simulink model "dspace_2019"  (R2019b)
settings: Solver=FixedStepDiscrete  StartTime=0.0  StopTime=Inf  FixedStep=1e-3  RelTol=1e-3
PostLoadFcn:
  | , if any(exist('dsrtsu_mdlpostloadfcn', 'file') ~= 0), dsrtsu_mdlpostloadfcn('Execute', bdroot); end,
undefined symbols (not defined in the file): ami, amk1_setpoints_1, amk2_setpoints_1, amk3_setpoints_1, amk4_setpoints_1, as, digital, ebs, indicator, mcu_set_dbu_indicator_points, mcu_set_ecu_indicator_points, res_ntm_node_control
libraries: rtican x63, simulink x5, rti1401lib_dio_type3 x4, simulink_extras x1
(part 3 of 16)

== system dspace_2019/GPIO TX ==
  tx_gpio4 : Inport  PortName=tx_gpio  Element=enable_inverter4
  tx_gpio1 : Inport  PortName=tx_gpio  Element=enable_inverter1
  tx_gpio2 : Inport  PortName=tx_gpio  Element=enable_inverter2
  tx_gpio3 : Inport  PortName=tx_gpio  Element=enable_inverter3
  DIO_TYPE3_BIT_OUT_CH_BL1 : rti1401lib_dio_type3/DIO_TYPE3_BIT_OUT_CH_BL1  DSProperties=struct('RTI',struct('Version',uint32(2),'BlockType',struct('isSLSource',uint8(0),'isSLSink',uint8(1),'isHWSource',uint8(0),'isHWSink',uint8(1),'isSetup',uint8(0),'isInline',uint8(1),'isNonInline',uint8(0),'isInterrupt',uint8(0),'isChannelwise',uint8(1)),'IOBoardType',{{'DS1401','STD','DIOT3'}},'UnitType','BIT','Identifier','BITOUTCH','DialogType','ML','BlockSet','NONE','SlaveProcessor','NONE'))  RTIBlockInterface=struct('InputPortsWidth',int32(1),'InputPortsActive',1,'InputPortsDataType',{{'SS_BOOLEAN'}},'InputPortsName',{{'In'}},'BlockDisplay',{{['DIO TP3 BIT OUT\n Channelwise\nModule: 1\nPort: 1\nChannel: 2'],'center'}},'IconTransparency','on','InitLevel',3,'DialogFcn','rti1401stddiot3bitoutchgui','BlockName',struct('Token',{{'DIO_TYPE3_BIT_OUT_CH_BL1'}}))  RTIBlockParameters=struct('ModuleNo',{{1,'OFF',[1 16]}},'PortNo',{{1,'OFF',[1 3]}},'ChannelNo',{{2,'OFF',[1 16]}},'OutputStateInit',{{0,'OFF',[0 1]}},'TerminationMode',{{0,'OFF',[0 1]}},'OutputStateTermValidate',{{0,'OFF',[0 1]}},'OutputStateTerm',{{0,'OFF',[0 1]}},'SupplyRailsCh',{{[1 1],'OFF',[0 1 0 1]}},'TLCFileName',{{'rti1401dio_t3_bit_out_ch','OFF',[]}},'EnableInterrupt',{{0,'OFF',[0 1]}},'TriggerEdgeType',{{1,'OFF',[1 3]}})  RTISFcnParameters=struct('ModuleNo','int32','PortNo','int16','ChannelNo','int16','SupplyRailsCh','int16','OutputStateInit','int16','TerminationMode','int16','OutputStateTermValidate','int16','OutputStateTerm','int16','TLCFileName','char','EnableInterrupt','int16','TriggerEdgeType','int32')  RTIBlockParaDefault=struct('ModuleNo',1,'PortNo',1,'ChannelNo',1,'OutputStateInit',0,'TerminationMode',0,'OutputStateTermValidate',0,'OutputStateTerm',0,'SupplyRailsCh',[1 1],'TLCFileName','rti1401dio_t3_bit_out_ch','EnableInterrupt',0,'TriggerEdgeType',1)
  DIO_TYPE3_BIT_OUT_CH_BL2 : rti1401lib_dio_type3/DIO_TYPE3_BIT_OUT_CH_BL1  DSProperties=struct('RTI',struct('Version',uint32(2),'BlockType',struct('isSLSource',uint8(0),'isSLSink',uint8(1),'isHWSource',uint8(0),'isHWSink',uint8(1),'isSetup',uint8(0),'isInline',uint8(1),'isNonInline',uint8(0),'isInterrupt',uint8(0),'isChannelwise',uint8(1)),'IOBoardType',{{'DS1401','STD','DIOT3'}},'UnitType','BIT','Identifier','BITOUTCH','DialogType','ML','BlockSet','NONE','SlaveProcessor','NONE'))  RTIBlockInterface=struct('InputPortsWidth',int32(1),'InputPortsActive',1,'InputPortsDataType',{{'SS_BOOLEAN'}},'InputPortsName',{{'In'}},'BlockDisplay',{{['DIO TP3 BIT OUT\n Channelwise\nModule: 1\nPort: 1\nChannel: 3'],'center'}},'IconTransparency','on','InitLevel',3,'DialogFcn','rti1401stddiot3bitoutchgui','BlockName',struct('Token',{{'DIO_TYPE3_BIT_OUT_CH_BL1'}}))  RTIBlockParameters=struct('ModuleNo',{{1,'OFF',[1 16]}},'PortNo',{{1,'OFF',[1 3]}},'ChannelNo',{{3,'OFF',[1 16]}},'OutputStateInit',{{0,'OFF',[0 1]}},'TerminationMode',{{0,'OFF',[0 1]}},'OutputStateTermValidate',{{0,'OFF',[0 1]}},'OutputStateTerm',{{0,'OFF',[0 1]}},'SupplyRailsCh',{{[1 1],'OFF',[0 1 0 1]}},'TLCFileName',{{'rti1401dio_t3_bit_out_ch','OFF',[]}},'EnableInterrupt',{{0,'OFF',[0 1]}},'TriggerEdgeType',{{1,'OFF',[1 3]}})  RTISFcnParameters=struct('ModuleNo','int32','PortNo','int16','ChannelNo','int16','SupplyRailsCh','int16','OutputStateInit','int16','TerminationMode','int16','OutputStateTermValidate','int16','OutputStateTerm','int16','TLCFileName','char','EnableInterrupt','int16','TriggerEdgeType','int32')  RTIBlockParaDefault=struct('ModuleNo',1,'PortNo',1,'ChannelNo',1,'OutputStateInit',0,'TerminationMode',0,'OutputStateTermValidate',0,'OutputStateTerm',0,'SupplyRailsCh',[1 1],'TLCFileName','rti1401dio_t3_bit_out_ch','EnableInterrupt',0,'TriggerEdgeType',1)
  DIO_TYPE3_BIT_OUT_CH_BL3 : rti1401lib_dio_type3/DIO_TYPE3_BIT_OUT_CH_BL1  DSProperties=struct('RTI',struct('Version',uint32(2),'BlockType',struct('isSLSource',uint8(0),'isSLSink',uint8(1),'isHWSource',uint8(0),'isHWSink',uint8(1),'isSetup',uint8(0),'isInline',uint8(1),'isNonInline',uint8(0),'isInterrupt',uint8(0),'isChannelwise',uint8(1)),'IOBoardType',{{'DS1401','STD','DIOT3'}},'UnitType','BIT','Identifier','BITOUTCH','DialogType','ML','BlockSet','NONE','SlaveProcessor','NONE'))  RTIBlockInterface=struct('InputPortsWidth',int32(1),'InputPortsActive',1,'InputPortsDataType',{{'SS_BOOLEAN'}},'InputPortsName',{{'In'}},'BlockDisplay',{{['DIO TP3 BIT OUT\n Channelwise\nModule: 1\nPort: 1\nChannel: 4'],'center'}},'IconTransparency','on','InitLevel',3,'DialogFcn','rti1401stddiot3bitoutchgui','BlockName',struct('Token',{{'DIO_TYPE3_BIT_OUT_CH_BL1'}}))  RTIBlockParameters=struct('ModuleNo',{{1,'OFF',[1 16]}},'PortNo',{{1,'OFF',[1 3]}},'ChannelNo',{{4,'OFF',[1 16]}},'OutputStateInit',{{0,'OFF',[0 1]}},'TerminationMode',{{0,'OFF',[0 1]}},'OutputStateTermValidate',{{0,'OFF',[0 1]}},'OutputStateTerm',{{0,'OFF',[0 1]}},'SupplyRailsCh',{{[1 1],'OFF',[0 1 0 1]}},'TLCFileName',{{'rti1401dio_t3_bit_out_ch','OFF',[]}},'EnableInterrupt',{{0,'OFF',[0 1]}},'TriggerEdgeType',{{1,'OFF',[1 3]}})  RTISFcnParameters=struct('ModuleNo','int32','PortNo','int16','ChannelNo','int16','SupplyRailsCh','int16','OutputStateInit','int16','TerminationMode','int16','OutputStateTermValidate','int16','OutputStateTerm','int16','TLCFileName','char','EnableInterrupt','int16','TriggerEdgeType','int32')  RTIBlockParaDefault=struct('ModuleNo',1,'PortNo',1,'ChannelNo',1,'OutputStateInit',0,'TerminationMode',0,'OutputStateTermValidate',0,'OutputStateTerm',0,'SupplyRailsCh',[1 1],'TLCFileName','rti1401dio_t3_bit_out_ch','EnableInterrupt',0,'TriggerEdgeType',1)
  DIO_TYPE3_BIT_OUT_CH_BL4 : rti1401lib_dio_type3/DIO_TYPE3_BIT_OUT_CH_BL1  DSProperties=struct('RTI',struct('Version',uint32(2),'BlockType',struct('isSLSource',uint8(0),'isSLSink',uint8(1),'isHWSource',uint8(0),'isHWSink',uint8(1),'isSetup',uint8(0),'isInline',uint8(1),'isNonInline',uint8(0),'isInterrupt',uint8(0),'isChannelwise',uint8(1)),'IOBoardType',{{'DS1401','STD','DIOT3'}},'UnitType','BIT','Identifier','BITOUTCH','DialogType','ML','BlockSet','NONE','SlaveProcessor','NONE'))  RTIBlockInterface=struct('InputPortsWidth',int32(1),'InputPortsActive',1,'InputPortsDataType',{{'SS_BOOLEAN'}},'InputPortsName',{{'In'}},'BlockDisplay',{{['DIO TP3 BIT OUT\n Channelwise\nModule: 1\nPort: 1\nChannel: 1'],'center'}},'IconTransparency','on','InitLevel',3,'DialogFcn','rti1401stddiot3bitoutchgui','BlockName',struct('Token',{{'DIO_TYPE3_BIT_OUT_CH_BL1'}}))  RTIBlockParameters=struct('ModuleNo',{{1,'OFF',[1 16]}},'PortNo',{{1,'OFF',[1 3]}},'ChannelNo',{{1,'OFF',[1 16]}},'OutputStateInit',{{0,'OFF',[0 1]}},'TerminationMode',{{0,'OFF',[0 1]}},'OutputStateTermValidate',{{0,'OFF',[0 1]}},'OutputStateTerm',{{0,'OFF',[0 1]}},'SupplyRailsCh',{{[1 1],'OFF',[0 1 0 1]}},'TLCFileName',{{'rti1401dio_t3_bit_out_ch','OFF',[]}},'EnableInterrupt',{{0,'OFF',[0 1]}},'TriggerEdgeType',{{1,'OFF',[1 3]}})  RTISFcnParameters=struct('ModuleNo','int32','PortNo','int16','ChannelNo','int16','SupplyRailsCh','int16','OutputStateInit','int16','TerminationMode','int16','OutputStateTermValidate','int16','OutputStateTerm','int16','TLCFileName','char','EnableInterrupt','int16','TriggerEdgeType','int32')  RTIBlockParaDefault=struct('ModuleNo',1,'PortNo',1,'ChannelNo',1,'OutputStateInit',0,'TerminationMode',0,'OutputStateTermValidate',0,'OutputStateTerm',0,'SupplyRailsCh',[1 1],'TLCFileName','rti1401dio_t3_bit_out_ch','EnableInterrupt',0,'TriggerEdgeType',1)
  wires:
  tx_gpio1/1 -> DIO_TYPE3_BIT_OUT_CH_BL4/1
  tx_gpio4/1 -> DIO_TYPE3_BIT_OUT_CH_BL3/1
  tx_gpio3/1 -> DIO_TYPE3_BIT_OUT_CH_BL2/1
  tx_gpio2/1 -> DIO_TYPE3_BIT_OUT_CH_BL1/1

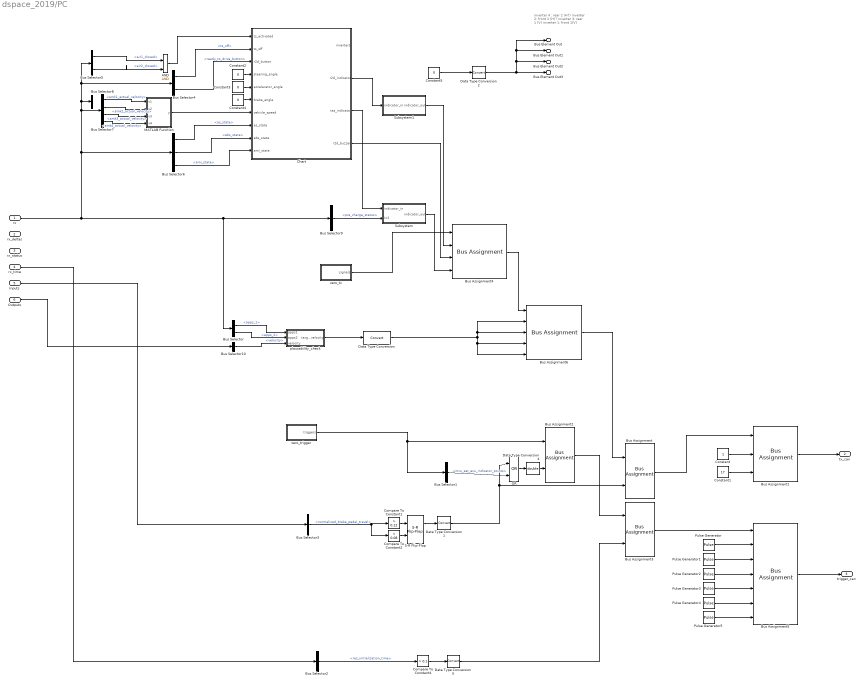
== system dspace_2019/PC ==
  note: inverter 4 : rear 2 (H?)
      | inverter 2: front 2 (H)?
      | inverter 3: rear 1 (V)
      | inverter 1: front 1(V)
  rx : Inport
  rx_deltas : Inport  Port=2
  rx_status : Inport  Port=3
  rx_time : Inport  Port=4
  Inputs : Inport  Port=5
  Outputs : Inport  Port=6
  AND : Logic  IconShape=distinctive  AllPortsSameDT=off  OutDataTypeStr=boolean
  Bus Assignment : BusAssignment  AssignedSignals=mcu_set_ecu_indicator_points.brake_light
  Bus Assignment1 : BusAssignment  AssignedSignals=res_ntm_node_control.requested_state,res_ntm_node_control.node_id
  Bus Assignment2 : BusAssignment  AssignedSignals=mcu_set_ecu_indicator_points
  Bus Assignment3 : BusAssignment  AssignedSignals=res_ntm_node_control
  Bus Assignment4 : BusAssignment  AssignedSignals=mcu_set_dbu_indicator_points.r2d_indicator_on,mcu_set_ecu_indicator_points.r2d_sound,mcu_set_dbu_indicator_points.ts_indicator_on
  Bus Assignment5 : BusAssignment  AssignedSignals=mcu_set_ecu_indicator_points,mcu_set_dbu_indicator_points,amk1_setpoints_1,amk2_setpoints_1,amk3_setpoints_1,amk4_setpoints_1
  Bus Assignment6 : BusAssignment  AssignedSignals=amk1_setpoints_1.amk1_target_velocity,amk2_setpoints_1.amk2_target_velocity,amk3_setpoints_1.amk3_target_velocity,amk4_setpoints_1.amk4_target_velocity
  Bus Selector : BusSelector  OutputSignals=dcu_pps.apps_1,dcu_pps.apps_2
  Bus Selector1 : BusSelector  OutputSignals=mcu_set_ecu_indicator_points
  Bus Selector10 : BusSelector  OutputSignals=velocity
  Bus Selector2 : BusSelector  OutputSignals=res_initialization_time
  Bus Selector3 : BusSelector  OutputSignals=normalized_brake_pedal_travel
  Bus Selector4 : BusSelector  OutputSignals=ecu_status.ts_off,dbu_status_1.ready_to_drive_button
  Bus Selector5 : BusSelector  OutputSignals=ams_status_1.air1_closed,ams_status_1.air2_closed
  Bus Selector6 : BusSelector  OutputSignals=dv_system_status.as_state,dv_system_status.ebs_state,dv_system_status.ami_state
  Bus Selector7 : BusSelector  OutputSignals=amk1_actual_values_1.amk1_actual_velocity,amk2_actual_values_1.amk2_actual_velocity,amk3_actual_values_1.amk3_actual_velocity,amk4_actual_values_1.amk4_actual_velocity
  Bus Selector8 : BusSelector  OutputSignals=dv_system_status.steering_state
  Bus Selector9 : BusSelector  OutputSignals=ams_status_1.pre_charge_status
  Chart : Stateflow chart  TreatAsAtomicUnit=on
  Compare To Constant1 : simulink/Logic and Bit Operations/Compare To Constant  relop=>  const=0.12  OutDataTypeStr=boolean
  Compare To Constant2 : simulink/Logic and Bit Operations/Compare To Constant  relop=<  const=0.08  OutDataTypeStr=boolean
  Compare To Constant4 : simulink/Logic and Bit Operations/Compare To Constant  relop=>  const=0.1  OutDataTypeStr=boolean
  Constant : Constant
  Constant1 : Constant  Value=17
  Constant{2..5} (4 alike) : Constant  Value=0
  Data Type Conversion{,1..2,5} (4 alike) : DataTypeConversion
  Data Type Conversion4 : DataTypeConversion  OutDataTypeStr=double
  MATLAB Function : MATLAB Function  TreatAsAtomicUnit=on
  OR : Logic  Operator=OR  IconShape=distinctive  AllPortsSameDT=off  OutDataTypeStr=boolean
  Pulse Generator{,1..5} (6 alike) : DiscretePulseGenerator  PulseType=Time based  Period=0.02  PulseWidth=50
  S-R Flip-Flop : simulink_extras/Flip Flops/S-R Flip-Flop  initial_condition=0
  Subsystem : Subsystem
  Subsystem1 : Subsystem
  plausability_check : Subsystem
  zero_trigger : Subsystem
  "zero_tx " : Subsystem
  Bus Element Out : Outport  PortName=tx_gpio  Element=enable_inverter1
  Bus Element Out1 : Outport  PortName=tx_gpio  Element=enable_inverter2
  Bus Element Out2 : Outport  PortName=tx_gpio  Element=enable_inverter3
  Bus Element Out3 : Outport  PortName=tx_gpio  Element=enable_inverter4
  "tx_can " : Outport  Port=2
  trigger_can : Outport  Port=3
  wires:
  Data Type Conversion1/1 -> OR/1, Bus Assignment/2
  S-R Flip-Flop/1 -> Data Type Conversion1/1
  Compare To Constant1/1 -> S-R Flip-Flop/1
  Compare To Constant2/1 -> S-R Flip-Flop/2
  rx_time/1 -> Bus Selector2/1
  Constant5/1 -> Data Type Conversion2/1
  Bus Assignment/1 -> Bus Assignment1/1
  Bus Assignment1/1 -> "tx_can "/1
  Constant/1 -> Bus Assignment1/2
  Constant1/1 -> Bus Assignment1/3
  zero_trigger/1(triggers) -> Bus Selector1/1, Bus Assignment2/1
  Bus Assignment2/1 -> Bus Assignment3/1
  Bus Selector1/1 -> OR/2  "<mcu_set_ecu_indicator_points>"
  Bus Assignment3/1 -> Bus Assignment5/1
  OR/1 -> Data Type Conversion4/1
  Data Type Conversion4/1 -> Bus Assignment2/2
  Bus Selector2/1 -> Compare To Constant4/1  "<res_initialization_time>"
  Data Type Conversion5/1 -> Bus Assignment3/2
  Compare To Constant4/1 -> Data Type Conversion5/1
  Bus Selector3/1 -> Compare To Constant1/1, Compare To Constant2/1  "<normalized_brake_pedal_travel>"
  Inputs/1 -> Bus Selector3/1
  Bus Selector7/3 -> MATLAB Function/3(v3)  "<amk3_actual_velocity>"
  Chart/3(tsa_indicator) -> Subsystem/1(indicator_in)
  Constant3/1 -> Chart/5(accelerator_angle)
  Chart/4(r2d_buzzer) -> Bus Assignment4/3
  MATLAB Function/1(y) -> Chart/7(vehicle_speed)
  Bus Selector6/2 -> Chart/9(ebs_state)  "<ebs_state>"
  Constant2/1 -> Chart/4(steering_angle)
  Bus Selector6/1 -> Chart/8(as_state)  "<as_state>"
  Chart/2(r2d_indicator) -> Subsystem1/1(indicator_in)
  Bus Selector6/3 -> Chart/10(ami_state)  "<ami_state>"
  Bus Selector5/1 -> AND/1  "<air1_closed>"
  Subsystem1/1(indicator_out) -> Bus Assignment4/2
  Bus Selector7/4 -> MATLAB Function/4(v4)  "<amk4_actual_velocity>"
  rx/1 -> Bus Selector5/1, Bus Selector4/1, Bus Selector8/1, Bus Selector7/1, Bus Selector6/1, Bus Selector9/1, Bus Selector/1
  Bus Selector5/2 -> AND/2  "<air2_closed>"
  Bus Selector4/1 -> Chart/2(ts_off)  "<ts_off>"
  Bus Selector4/2 -> Chart/3(r2d_button)  "<ready_to_drive_button>"
  Bus Selector7/2 -> MATLAB Function/2(v2)  "<amk2_actual_velocity>"
  Bus Selector9/1 -> Subsystem/2(In2)  "<pre_charge_status>"
  Bus Selector7/1 -> MATLAB Function/1(v1)  "<amk1_actual_velocity>"
  Subsystem/1(indicator_out) -> Bus Assignment4/4
  Constant4/1 -> Chart/6(brake_angle)
  AND/1 -> Chart/1(ts_activated)
  Bus Assignment5/1 -> trigger_can/1
  Pulse Generator3/1 -> Bus Assignment5/5
  Pulse Generator2/1 -> Bus Assignment5/4
  Pulse Generator/1 -> Bus Assignment5/2
  Pulse Generator4/1 -> Bus Assignment5/6
  Pulse Generator5/1 -> Bus Assignment5/7
  Pulse Generator1/1 -> Bus Assignment5/3
  "zero_tx "/1(signals) -> Bus Assignment4/1
  Data Type Conversion2/1 -> Bus Element Out/1, Bus Element Out1/1, Bus Element Out2/1, Bus Element Out3/1
  Bus Selector/1 -> plausability_check/1(apps1)  "<apps_1>"
  Bus Selector/2 -> plausability_check/2(apps2)  "<apps_2>"
  Bus Assignment4/1 -> Bus Assignment6/1
  Data Type Conversion/1 -> Bus Assignment6/5, Bus Assignment6/4, Bus Assignment6/3, Bus Assignment6/2
  Bus Assignment6/1 -> Bus Assignment/1
  Outputs/1 -> Bus Selector10/1
  Bus Selector10/1 -> plausability_check/3(velocity)  "<velocity>"
  plausability_check/1(target_velocity) -> Data Type Conversion/1

== system dspace_2019/RTI Data ==
  RTI Data Store : Subsystem  Tag="struct('private',struct('version',struct('dsVer',uint32(2),'dsVerCreation',uint32(2),'RTI',struct('ver','7.13','type','RTI1401')),'access',struct('type','Model','isPerm',1,'created',['29-Jun-2022 11:04:06'],'modified',['25-Jul-2022 13:04:18'],'location','')),'public',struct('main',struct('data',[]),'sub',struct('name',{{'dspace'}},'data',{{struct('TH',struct('thTaskInfo',struct('taskType',{'TIMER','HWINT','TMRINT','SWINT','GLINT'},'tasksNumOf',{1,0,0,0,0},'srcIds',{{'TIMERA'},{},{},{},{}},'taskNames',{{['Timer Task 1']},{},{},{},{}})),'th_tc',struct('dataType','TASK','taskGroupId','','taskGroupList',{{}},'taskSchedulingPolicy','FCFS','taskType','TIMER','blkh',-1,'srcId','TIMERA','srcSgnName',['Timer A interrupt'],'srcCpuName','','taskName',['Timer Task 1  [0.001] s'],'taskNameDisplayExt','','smplTime',0.001,'smplTimeOffs',0,'hasFixedPriority',0,'priority',1,'hasFixedOvc',0,'ovcType',1,'ovcMax',1),'tc_th',struct('dataType','TASK','taskGroupId','','taskGroupList',{{}},'taskSchedulingPolicy','FCFS','taskType','TIMER','blkh',-1,'srcId','TIMERA','srcSgnName',['Timer A interrupt'],'srcCpuName','','taskName',['Timer Task 1  [0.001] s'],'taskNameDisplayExt','','smplTime',0.001,'smplTimeOffs',0,'hasFixedPriority',0,'priority',1,'hasFixedOvc',0,'ovcType',1,'ovcMax',1))}})))"  mask(RTI_DATA_STORE){}
      mask help:
      | RTI Data Store Block. This block is used by RTI to store internal model dependent data. Deleting this block will result in data loss.
      |
      | NEVER DELETE, COPY, OR MODIFY THIS BLOCK!
      mask Help:
      | RTI Data Store Block. This block is used by RTI to store internal model dependent data. Deleting this block will result in data loss.
      | 
      | NEVER DELETE, COPY, OR MODIFY THIS BLOCK!
      mask Display: text(0.5, 0.5, ' ', 'HorizontalAlignment', 'center');

== system dspace_2019/Signal Preconditioning ==
  rx : Inport
  rx_deltas : Inport  Port=2
  rx_status : Inport  Port=3
  rx_time : Inport  Port=4
  Bus Selector8 : BusSelector  OutputSignals=dcu_pps.bpps_1,dcu_pps.bpps_2,dcu_pps.apps_1,dcu_pps.apps_2
  Compare To Constant : simulink/Logic and Bit Operations/Compare To Constant  relop=>  const=0.1  OutDataTypeStr=boolean
  Integrator : Integrator  ExternalReset=falling
  MATLAB Function1 : MATLAB Function  TreatAsAtomicUnit=on
  MATLAB Function2 : MATLAB Function  TreatAsAtomicUnit=on
  Bus Element Out : Outport  PortName=Inputs  Element=normalized_brake_pedal_travel
  Out Bus Element : Outport  PortName=Inputs  Element=apps_implausability
  Out Bus Element1 : Outport  PortName=Inputs  Element=normalized_accelerator_pedal_travel
  wires:
  Bus Selector8/2 -> MATLAB Function1/2(bpps2)  "<bpps_2>"
  Bus Selector8/1 -> MATLAB Function1/1(bpps1)  "<bpps_1>"
  rx/1 -> Bus Selector8/1
  MATLAB Function1/1(normalized_brake_pedal_travel) -> Bus Element Out/1
  Bus Selector8/3 -> MATLAB Function2/1(apps1)  "<apps_1>"
  Bus Selector8/4 -> MATLAB Function2/2(apps2)  "<apps_2>"
  MATLAB Function2/2(implausability) -> Integrator/2, Integrator/1
  Integrator/1 -> Compare To Constant/1
  Compare To Constant/1 -> Out Bus Element/1
  MATLAB Function2/1(normalized_accelerator_pedal_travel) -> Out Bus Element1/1

== system dspace_2019/Vehicular Control ==
  rx : Inport
  Bus Element In : Inport  Port=2  PortName=Inputs  Element=normalized_brake_pedal_travel
  In Bus Element : Inport  Port=2  PortName=Inputs  Element=normalized_accelerator_pedal_travel
  Bus Selector : BusSelector  OutputSignals=dv_system_status.as_state,dv_control_target.dv_speed_target
  MATLAB Function : MATLAB Function  TreatAsAtomicUnit=on
  Out Bus Element : Outport  PortName=Outputs  Element=velocity
  wires:
  rx/1 -> Bus Selector/1
  Bus Selector/1 -> MATLAB Function/1(car_state)  "<as_state>"
  In Bus Element/1 -> MATLAB Function/3(accelerator_pedal)
  Bus Selector/2 -> MATLAB Function/2(as_speed)  "<dv_speed_target>"
  MATLAB Function/1(velocity) -> Out Bus Element/1

== system dspace_2019/CAN RX/FSE_EnergyMeter_Data ==
  FSE_EnergyMeter_Data1 : rtican/RTICAN Receive (RX)   Reserved1=[]  Reserved2=[]  Reserved3=[]  Reserved4=[]  SfcnMessage=[]  Msg_Struct=[]  BoardTypeNo=[]  BoardNo=[]  ChannelNo=[]  Parameters=[]  DialogFcn=[]  UnitName=[]  Revision=[]  UnitValues=[]  DSProperties=struct('RTI',struct('Version',uint32(5),'BlockType',struct('isSLSource',uint8(1),'isSLSink',uint8(1),'isHWSource',uint8(0),'isHWSink',uint8(0),'isSetup',uint8(0),'isInline',uint8(1),'isNonInline',uint8(0),'isInterrupt',uint8(0),'isChannelwise',uint8(0)),'IOBoardType','RTICAN','UnitType','MESSAGE','Identifier','RX','DialogType','MSVC','BlockSet','RTICAN','SlaveProcessor','CAN'))  RTIBlockInterface=struct('OutputPortsWidth',int32([1 1 1 1 1 1 1 1]),'OutputPortsActive',[1 1 1 1 1 1 1 1],'OutputPortsName',{{'MsgCntr','Status','Power','Voltage','Current',['RX status'],['RX time'],['RX delta time']}},'OutputPortsDataType',{{'SS_DOUBLE','SS_DOUBLE','SS_DOUBLE','SS_DOUBLE','SS_DOUBLE','SS_DOUBLE','SS_DOUBLE','SS_DOUBLE'}},'OutputPortsLabel',{{'MsgCntr','Status','Power','Voltage','Current','','',''}},'OutputPortsLabelMode','ON','InputPortsWidth',int32(0),'InputPortsActive',0,'DialogFcn','rtican_message_interface_gui','BlockDisplay',{{'','center'}},'IconTransparency','on','ParameterTunableNames',{{}},'InitLevel',3,'BlockName',struct('Token',{{'FSE_EnergyMeter_Data'}}),'SampleTime',{{-1}},'TriggerPort',{{'none'}},'EnablePort',{{'none'}})  RTIBlockParameters=struct('BoardTypeNo',{{1,'OFF',[]}},'BoardNo',{{1,'ON',[1 16]}},'ChannelNo',{{2,'ON',[1 2]}},'Parameters',{{struct('DataFileSupport',struct('DataFileSelectedMaster',1,'DataFileSelectedLocal',1,'DataFileName','c:\users\oscar\documents\github\sw_infrastructure\kthfspe_python\databases\can1.dbc|','DataFileDate',{{{['10-Jul-2022 16:14:04']}}},'SelectedFile','c:\users\oscar\documents\github\sw_infrastructure\kthfspe_python\databases\can1.dbc'),'Options',struct('StatusSelected',1,'TimeSelected',1,'DeltaTimeSelected',1,'BytePortSelected',0,'MessageLengthSelected',0,'TriggerPort',struct('Selected',0,'TriggerType',0),'UserCoding',struct('Selected',0,'InterfaceFile','UserDecodingFile','FcnName','UserDecodeFcn','InportSelected',0,'InportWidth',1,'OutportSelected',0,'OutportWidth',1),'EnablePortSelected',0,'SignalOnPortnameSelected',1,'UseRXService',0),'Message',struct('MsgOnBlocknameSelected',1,'MsgName','FSE_EnergyMeter_Data','MsgIdFormat',0,'MsgId',1072,'MsgLength',8,'NumSignals',5,'SampleTime',-1,'Signal',struct('SgnName',{'MsgCntr','Status','Power','Voltage','Current'},'SgnStartBit',{0,8,16,32,48},'SgnLength',{8,8,16,16,16},'SgnType',{0,0,0,0,0},'ModeValue',{-1,-1,-1,-1,-1},'DataType',{0,0,1,1,1},'ByteLayout',{0,0,0,0,0},'Factor',{1,1,3,0.04,0.05},'Offset',{0,0,0,0,0},'SgnComment',{{''},{''},{''},{''},{''}},'SgnUnit',{'','','W','V','A'},'Min',{0,0,-98304,-1310.72,-1638.4},'Max',{255,255,98301,1310.68,1638.35},'SLDataType',{'SS_DOUBLE','SS_DOUBLE','SS_DOUBLE','SS_DOUBLE','SS_DOUBLE'}),'MsgIdNumFormat',0,'MsgComment',{{''}}),'Version',1.2,'general',struct('isFromLib',0)),'OFF',[]}},'GroupId',{{struct('Group',{{'RTICAN'}},'No',1,'Behavior',{{'NAMECHANGE'}},'BlockType',{{'SINK'}},'NameChangeFlag',0),'OFF',[]}},'SFcnRTICANMessage',{{struct('MsgType','RX','SFcnPortType','Scalar','MsgName','FSE_EnergyMeter_Data','MsgIdFormat','STD','MsgId',1072,'MsgLength',8,'NumSignals',5,'SampleTime',-1,'Signal',struct('SgnName',{'MsgCntr','Status','Power','Voltage','Current'},'SgnStartBit',{0,8,16,32,48},'SgnLength',{8,8,16,16,16},'SgnType',{'standard','standard','standard','standard','standard'},'ModeValue',{-1,-1,-1,-1,-1},'DataType',{['unsigned int'],['unsigned int'],['signed int'],['signed int'],['signed int']},'ByteLayout',{['little endian'],['little endian'],['little endian'],['little endian'],['little endian']},'Factor',{1,1,3,0.04,0.05},'Offset',{0,0,0,0,0},'SLDataType',{'SS_DOUBLE','SS_DOUBLE','SS_DOUBLE','SS_DOUBLE','SS_DOUBLE'}),'StatusSelected','yes','TimeSelected','yes','DeltaTimeSelected','yes','BytePortSelected','no','MessageLengthSelected','no','TriggerPort',struct('Selected','no','TriggerType',0),'UserCoding',struct('Selected','no','InterfaceFile','UserDecodingFile','FcnName','UserDecodeFcn','InportSelected','no','InportWidth',1,'OutportSelected','no','OutportWidth',1),'EnablePortSelected','no','UseRXService','no','BoardType','DS1','BoardNo',1,'ControllerNo',1),'OFF',[]}},'TLCFileName',{{'rtican_rx_message','OFF',[]}})  RTISFcnParameters=struct('SFcnRTICANMessage','struct','TLCFileName','char')  RTIBlockParaDefault=struct('BoardTypeNo',4302,'BoardNo',1,'ChannelNo',1,'Parameters',struct('DataFileSupport',struct('DataFileSelectedMaster',0,'DataFileSelectedLocal',0,'DataFileName','','DataFileDate','','SelectedFile',['<no file selected>']),'Options',struct('StatusSelected',1,'TimeSelected',1,'DeltaTimeSelected',1,'BytePortSelected',0,'MessageLengthSelected',0,'TriggerPort',struct('Selected',0,'TriggerType','rising'),'UserCoding',struct('Selected',0,'InterfaceFile','UserDecodingFile','FcnName','UserDecodeFcn','InportSelected',0,'InportWidth',1,'OutportSelected',0,'OutportWidth',1),'EnablePortSelected',0,'SignalOnPortnameSelected',1,'UseRXService',0),'Message',struct('MsgOnBlocknameSelected',0,'MsgName',['RX Message'],'MsgIdFormat',0,'MsgId',100,'MsgLength',8,'NumSignals',1,'SampleTime',-1,'Signal',struct('SgnName',['RX signal'],'SgnStartBit',0,'SgnLength',8,'SgnType',0,'ModeValue',-1,'DataType',0,'SLDataType','SS_DOUBLE','ByteLayout',0,'Factor',1,'Offset',0,'Min',0,'Max',255,'SgnComment',{{}},'SgnUnit',''),'MsgIdNumFormat',0,'MsgComment',{{''}}),'Version',1.2,'general',struct('isFromLib',1)),'GroupId',struct('Group',{{'RTICAN'}},'No',1,'Behavior',{{'NAMECHANGE'}},'BlockType',{{'SINK'}},'NameChangeFlag',0),'SFcnRTICANMessage',struct('MsgType','RX','MsgName',['RX Message'],'MsgIdFormat','STD','MsgId',100,'MsgLength',8,'NumSignals',1,'SampleTime',-1,'Signal',struct('SgnName',['RX signal'],'SgnStartBit',0,'SgnLength',8,'SgnType','standard','ModeValue',-1,'DataType',['unsigned int'],'ByteLayout',['little endian'],'SLDataType','SS_DOUBLE','Factor',1,'Offset',0),'StatusSelected','yes','TimeSelected','yes','DeltaTimeSelected','yes','BytePortSelected','no','MessageLengthSelected','no','EnablePortSelected','no','UserCoding',struct('Selected','no','InterfaceFile','UserDecodingFile','FcnName','UserDecodeFcn','InportSelected','no','InportWidth',1,'OutportSelected','no','OutportWidth',1),'TriggerPort',struct('Selected','no','TriggerType','rising'),'UseRXService','no','BoardType','DS4302','BoardNo',1,'ControllerNo',1,'SFcnPortType','Scalar'),'TLCFileName','rtican_rx_message')
      settings: AttributesFormatString=Group Id: RTICAN1\n  SourceProductName=dSPACE RTI CAN Blockset
  clock_time : Clock
  sub_time : Sum  Inputs=+-
  MsgCntr_bus : Outport  PortName=signals  Element=MsgCntr
  Status_bus : Outport  PortName=signals  Element=Status
  Power_bus : Outport  PortName=signals  Element=Power
  Voltage_bus : Outport  PortName=signals  Element=Voltage
  Current_bus : Outport  PortName=signals  Element=Current
  status : Outport  Port=2
  time : Outport  Port=3
  delta : Outport  Port=4
  wires:
  clock_time/1 -> sub_time/1
  sub_time/1 -> time/1
  FSE_EnergyMeter_Data1/6 -> status/1
  FSE_EnergyMeter_Data1/7 -> sub_time/2
  FSE_EnergyMeter_Data1/8 -> delta/1
  FSE_EnergyMeter_Data1/1 -> MsgCntr_bus/1  "MsgCntr"
  FSE_EnergyMeter_Data1/2 -> Status_bus/1  "Status"
  FSE_EnergyMeter_Data1/3 -> Power_bus/1  "Power"
  FSE_EnergyMeter_Data1/4 -> Voltage_bus/1  "Voltage"
  FSE_EnergyMeter_Data1/5 -> Current_bus/1  "Current"

== system dspace_2019/CAN RX/SBG_ECAN_MSG_AUTO_SLIP_CURV ==
  SBG_ECAN_MSG_AUTO_SLIP_CURV1 : rtican/RTICAN Receive (RX)   Reserved1=[]  Reserved2=[]  Reserved3=[]  Reserved4=[]  SfcnMessage=[]  Msg_Struct=[]  BoardTypeNo=[]  BoardNo=[]  ChannelNo=[]  Parameters=[]  DialogFcn=[]  UnitName=[]  Revision=[]  UnitValues=[]  DSProperties=struct('RTI',struct('Version',uint32(5),'BlockType',struct('isSLSource',uint8(1),'isSLSink',uint8(1),'isHWSource',uint8(0),'isHWSink',uint8(0),'isSetup',uint8(0),'isInline',uint8(1),'isNonInline',uint8(0),'isInterrupt',uint8(0),'isChannelwise',uint8(0)),'IOBoardType','RTICAN','UnitType','MESSAGE','Identifier','RX','DialogType','MSVC','BlockSet','RTICAN','SlaveProcessor','CAN'))  RTIBlockInterface=struct('OutputPortsWidth',int32([1 1 1 1 1 1 1]),'OutputPortsActive',[1 1 1 1 1 1 1],'OutputPortsName',{{'ANGLE_TRACK','ANGLE_SLIP','CURVATURE_RADIUS','AUTO_STATUS',['RX status'],['RX time'],['RX delta time']}},'OutputPortsDataType',{{'SS_DOUBLE','SS_DOUBLE','SS_DOUBLE','SS_DOUBLE','SS_DOUBLE','SS_DOUBLE','SS_DOUBLE'}},'OutputPortsLabel',{{'ANGLE_TRACK','ANGLE_SLIP','CURVATURE_RADIUS','AUTO_STATUS','','',''}},'OutputPortsLabelMode','ON','InputPortsWidth',int32(0),'InputPortsActive',0,'DialogFcn','rtican_message_interface_gui','BlockDisplay',{{'','center'}},'IconTransparency','on','ParameterTunableNames',{{}},'InitLevel',3,'BlockName',struct('Token',{{'SBG_ECAN_MSG_AUTO_SLIP_CURV'}}),'SampleTime',{{-1}},'TriggerPort',{{'none'}},'EnablePort',{{'none'}})  RTIBlockParameters=struct('BoardTypeNo',{{1,'OFF',[]}},'BoardNo',{{1,'ON',[1 16]}},'ChannelNo',{{2,'ON',[1 2]}},'Parameters',{{struct('DataFileSupport',struct('DataFileSelectedMaster',1,'DataFileSelectedLocal',1,'DataFileName','c:\users\oscar\documents\github\sw_infrastructure\kthfspe_python\databases\can1.dbc|','DataFileDate',{{{['10-Jul-2022 16:14:04']}}},'SelectedFile','c:\users\oscar\documents\github\sw_infrastructure\kthfspe_python\databases\can1.dbc'),'Options',struct('StatusSelected',1,'TimeSelected',1,'DeltaTimeSelected',1,'BytePortSelected',0,'MessageLengthSelected',0,'TriggerPort',struct('Selected',0,'TriggerType',0),'UserCoding',struct('Selected',0,'InterfaceFile','UserDecodingFile','FcnName','UserDecodeFcn','InportSelected',0,'InportWidth',1,'OutportSelected',0,'OutportWidth',1),'EnablePortSelected',0,'SignalOnPortnameSelected',1,'UseRXService',0),'Message',struct('MsgOnBlocknameSelected',1,'MsgName','SBG_ECAN_MSG_AUTO_SLIP_CURV','MsgIdFormat',0,'MsgId',544,'MsgLength',7,'NumSignals',4,'SampleTime',-1,'Signal',struct('SgnName',{'ANGLE_TRACK','ANGLE_SLIP','CURVATURE_RADIUS','AUTO_STATUS'},'SgnStartBit',{0,16,32,48},'SgnLength',{16,16,16,8},'SgnType',{0,0,0,0},'ModeValue',{-1,-1,-1,-1},'DataType',{1,1,0,0},'ByteLayout',{0,0,0,0},'Factor',{0.0001,0.0001,0.01,1},'Offset',{0,0,0,0},'SgnComment',{{''},{''},{''},{''}},'SgnUnit',{'rad','rad','m',''},'Min',{-3.2768,-3.2768,0,0},'Max',{3.2767,3.2767,655.35,255},'SLDataType',{'SS_DOUBLE','SS_DOUBLE','SS_DOUBLE','SS_DOUBLE'}),'MsgIdNumFormat',0,'MsgComment',{{''}}),'Version',1.2,'general',struct('isFromLib',0)),'OFF',[]}},'GroupId',{{struct('Group',{{'RTICAN'}},'No',1,'Behavior',{{'NAMECHANGE'}},'BlockType',{{'SINK'}},'NameChangeFlag',0),'OFF',[]}},'SFcnRTICANMessage',{{struct('MsgType','RX','SFcnPortType','Scalar','MsgName','SBG_ECAN_MSG_AUTO_SLIP_CURV','MsgIdFormat','STD','MsgId',544,'MsgLength',7,'NumSignals',4,'SampleTime',-1,'Signal',struct('SgnName',{'ANGLE_TRACK','ANGLE_SLIP','CURVATURE_RADIUS','AUTO_STATUS'},'SgnStartBit',{0,16,32,48},'SgnLength',{16,16,16,8},'SgnType',{'standard','standard','standard','standard'},'ModeValue',{-1,-1,-1,-1},'DataType',{['signed int'],['signed int'],['unsigned int'],['unsigned int']},'ByteLayout',{['little endian'],['little endian'],['little endian'],['little endian']},'Factor',{0.0001,0.0001,0.01,1},'Offset',{0,0,0,0},'SLDataType',{'SS_DOUBLE','SS_DOUBLE','SS_DOUBLE','SS_DOUBLE'}),'StatusSelected','yes','TimeSelected','yes','DeltaTimeSelected','yes','BytePortSelected','no','MessageLengthSelected','no','TriggerPort',struct('Selected','no','TriggerType',0),'UserCoding',struct('Selected','no','InterfaceFile','UserDecodingFile','FcnName','UserDecodeFcn','InportSelected','no','InportWidth',1,'OutportSelected','no','OutportWidth',1),'EnablePortSelected','no','UseRXService','no','BoardType','DS1','BoardNo',1,'ControllerNo',1),'OFF',[]}},'TLCFileName',{{'rtican_rx_message','OFF',[]}})  RTISFcnParameters=struct('SFcnRTICANMessage','struct','TLCFileName','char')  RTIBlockParaDefault=struct('BoardTypeNo',4302,'BoardNo',1,'ChannelNo',1,'Parameters',struct('DataFileSupport',struct('DataFileSelectedMaster',0,'DataFileSelectedLocal',0,'DataFileName','','DataFileDate','','SelectedFile',['<no file selected>']),'Options',struct('StatusSelected',1,'TimeSelected',1,'DeltaTimeSelected',1,'BytePortSelected',0,'MessageLengthSelected',0,'TriggerPort',struct('Selected',0,'TriggerType','rising'),'UserCoding',struct('Selected',0,'InterfaceFile','UserDecodingFile','FcnName','UserDecodeFcn','InportSelected',0,'InportWidth',1,'OutportSelected',0,'OutportWidth',1),'EnablePortSelected',0,'SignalOnPortnameSelected',1,'UseRXService',0),'Message',struct('MsgOnBlocknameSelected',0,'MsgName',['RX Message'],'MsgIdFormat',0,'MsgId',100,'MsgLength',8,'NumSignals',1,'SampleTime',-1,'Signal',struct('SgnName',['RX signal'],'SgnStartBit',0,'SgnLength',8,'SgnType',0,'ModeValue',-1,'DataType',0,'SLDataType','SS_DOUBLE','ByteLayout',0,'Factor',1,'Offset',0,'Min',0,'Max',255,'SgnComment',{{}},'SgnUnit',''),'MsgIdNumFormat',0,'MsgComment',{{''}}),'Version',1.2,'general',struct('isFromLib',1)),'GroupId',struct('Group',{{'RTICAN'}},'No',1,'Behavior',{{'NAMECHANGE'}},'BlockType',{{'SINK'}},'NameChangeFlag',0),'SFcnRTICANMessage',struct('MsgType','RX','MsgName',['RX Message'],'MsgIdFormat','STD','MsgId',100,'MsgLength',8,'NumSignals',1,'SampleTime',-1,'Signal',struct('SgnName',['RX signal'],'SgnStartBit',0,'SgnLength',8,'SgnType','standard','ModeValue',-1,'DataType',['unsigned int'],'ByteLayout',['little endian'],'SLDataType','SS_DOUBLE','Factor',1,'Offset',0),'StatusSelected','yes','TimeSelected','yes','DeltaTimeSelected','yes','BytePortSelected','no','MessageLengthSelected','no','EnablePortSelected','no','UserCoding',struct('Selected','no','InterfaceFile','UserDecodingFile','FcnName','UserDecodeFcn','InportSelected','no','InportWidth',1,'OutportSelected','no','OutportWidth',1),'TriggerPort',struct('Selected','no','TriggerType','rising'),'UseRXService','no','BoardType','DS4302','BoardNo',1,'ControllerNo',1,'SFcnPortType','Scalar'),'TLCFileName','rtican_rx_message')
      settings: AttributesFormatString=Group Id: RTICAN1\n  SourceProductName=dSPACE RTI CAN Blockset
  clock_time : Clock
  sub_time : Sum  Inputs=+-
  ANGLE_TRACK_bus : Outport  PortName=signals  Element=ANGLE_TRACK
  ANGLE_SLIP_bus : Outport  PortName=signals  Element=ANGLE_SLIP
  CURVATURE_RADIUS_bus : Outport  PortName=signals  Element=CURVATURE_RADIUS
  AUTO_STATUS_bus : Outport  PortName=signals  Element=AUTO_STATUS
  status : Outport  Port=2
  time : Outport  Port=3
  delta : Outport  Port=4
  wires:
  clock_time/1 -> sub_time/1
  sub_time/1 -> time/1
  SBG_ECAN_MSG_AUTO_SLIP_CURV1/5 -> status/1
  SBG_ECAN_MSG_AUTO_SLIP_CURV1/6 -> sub_time/2
  SBG_ECAN_MSG_AUTO_SLIP_CURV1/7 -> delta/1
  SBG_ECAN_MSG_AUTO_SLIP_CURV1/1 -> ANGLE_TRACK_bus/1  "ANGLE_TRACK"
  SBG_ECAN_MSG_AUTO_SLIP_CURV1/2 -> ANGLE_SLIP_bus/1  "ANGLE_SLIP"
  SBG_ECAN_MSG_AUTO_SLIP_CURV1/3 -> CURVATURE_RADIUS_bus/1  "CURVATURE_RADIUS"
  SBG_ECAN_MSG_AUTO_SLIP_CURV1/4 -> AUTO_STATUS_bus/1  "AUTO_STATUS"

== system dspace_2019/CAN RX/SBG_ECAN_MSG_EKF_EULER ==
  SBG_ECAN_MSG_EKF_EULER1 : rtican/RTICAN Receive (RX)   Reserved1=[]  Reserved2=[]  Reserved3=[]  Reserved4=[]  SfcnMessage=[]  Msg_Struct=[]  BoardTypeNo=[]  BoardNo=[]  ChannelNo=[]  Parameters=[]  DialogFcn=[]  UnitName=[]  Revision=[]  UnitValues=[]  DSProperties=struct('RTI',struct('Version',uint32(5),'BlockType',struct('isSLSource',uint8(1),'isSLSink',uint8(1),'isHWSource',uint8(0),'isHWSink',uint8(0),'isSetup',uint8(0),'isInline',uint8(1),'isNonInline',uint8(0),'isInterrupt',uint8(0),'isChannelwise',uint8(0)),'IOBoardType','RTICAN','UnitType','MESSAGE','Identifier','RX','DialogType','MSVC','BlockSet','RTICAN','SlaveProcessor','CAN'))  RTIBlockInterface=struct('OutputPortsWidth',int32([1 1 1 1 1 1]),'OutputPortsActive',[1 1 1 1 1 1],'OutputPortsName',{{'ROLL','PITCH','YAW',['RX status'],['RX time'],['RX delta time']}},'OutputPortsDataType',{{'SS_DOUBLE','SS_DOUBLE','SS_DOUBLE','SS_DOUBLE','SS_DOUBLE','SS_DOUBLE'}},'OutputPortsLabel',{{'ROLL','PITCH','YAW','','',''}},'OutputPortsLabelMode','ON','InputPortsWidth',int32(0),'InputPortsActive',0,'DialogFcn','rtican_message_interface_gui','BlockDisplay',{{'','center'}},'IconTransparency','on','ParameterTunableNames',{{}},'InitLevel',3,'BlockName',struct('Token',{{'SBG_ECAN_MSG_EKF_EULER'}}),'SampleTime',{{-1}},'TriggerPort',{{'none'}},'EnablePort',{{'none'}})  RTIBlockParameters=struct('BoardTypeNo',{{1,'OFF',[]}},'BoardNo',{{1,'ON',[1 16]}},'ChannelNo',{{2,'ON',[1 2]}},'Parameters',{{struct('DataFileSupport',struct('DataFileSelectedMaster',1,'DataFileSelectedLocal',1,'DataFileName','c:\users\oscar\documents\github\sw_infrastructure\kthfspe_python\databases\can1.dbc|','DataFileDate',{{{['10-Jul-2022 16:14:04']}}},'SelectedFile','c:\users\oscar\documents\github\sw_infrastructure\kthfspe_python\databases\can1.dbc'),'Options',struct('StatusSelected',1,'TimeSelected',1,'DeltaTimeSelected',1,'BytePortSelected',0,'MessageLengthSelected',0,'TriggerPort',struct('Selected',0,'TriggerType',0),'UserCoding',struct('Selected',0,'InterfaceFile','UserDecodingFile','FcnName','UserDecodeFcn','InportSelected',0,'InportWidth',1,'OutportSelected',0,'OutportWidth',1),'EnablePortSelected',0,'SignalOnPortnameSelected',1,'UseRXService',0),'Message',struct('MsgOnBlocknameSelected',1,'MsgName','SBG_ECAN_MSG_EKF_EULER','MsgIdFormat',0,'MsgId',306,'MsgLength',6,'NumSignals',3,'SampleTime',-1,'Signal',struct('SgnName',{'ROLL','PITCH','YAW'},'SgnStartBit',{0,16,32},'SgnLength',{16,16,16},'SgnType',{0,0,0},'ModeValue',{-1,-1,-1},'DataType',{1,1,1},'ByteLayout',{0,0,0},'Factor',{0.0001,0.0001,0.0001},'Offset',{0,0,0},'SgnComment',{{''},{''},{''}},'SgnUnit',{'rad','rad','rad'},'Min',{-3.2768,-3.2768,-3.2768},'Max',{3.2767,3.2767,3.2767},'SLDataType',{'SS_DOUBLE','SS_DOUBLE','SS_DOUBLE'}),'MsgIdNumFormat',0,'MsgComment',{{''}}),'Version',1.2,'general',struct('isFromLib',0)),'OFF',[]}},'GroupId',{{struct('Group',{{'RTICAN'}},'No',1,'Behavior',{{'NAMECHANGE'}},'BlockType',{{'SINK'}},'NameChangeFlag',0),'OFF',[]}},'SFcnRTICANMessage',{{struct('MsgType','RX','SFcnPortType','Scalar','MsgName','SBG_ECAN_MSG_EKF_EULER','MsgIdFormat','STD','MsgId',306,'MsgLength',6,'NumSignals',3,'SampleTime',-1,'Signal',struct('SgnName',{'ROLL','PITCH','YAW'},'SgnStartBit',{0,16,32},'SgnLength',{16,16,16},'SgnType',{'standard','standard','standard'},'ModeValue',{-1,-1,-1},'DataType',{['signed int'],['signed int'],['signed int']},'ByteLayout',{['little endian'],['little endian'],['little endian']},'Factor',{0.0001,0.0001,0.0001},'Offset',{0,0,0},'SLDataType',{'SS_DOUBLE','SS_DOUBLE','SS_DOUBLE'}),'StatusSelected','yes','TimeSelected','yes','DeltaTimeSelected','yes','BytePortSelected','no','MessageLengthSelected','no','TriggerPort',struct('Selected','no','TriggerType',0),'UserCoding',struct('Selected','no','InterfaceFile','UserDecodingFile','FcnName','UserDecodeFcn','InportSelected','no','InportWidth',1,'OutportSelected','no','OutportWidth',1),'EnablePortSelected','no','UseRXService','no','BoardType','DS1','BoardNo',1,'ControllerNo',1),'OFF',[]}},'TLCFileName',{{'rtican_rx_message','OFF',[]}})  RTISFcnParameters=struct('SFcnRTICANMessage','struct','TLCFileName','char')  RTIBlockParaDefault=struct('BoardTypeNo',4302,'BoardNo',1,'ChannelNo',1,'Parameters',struct('DataFileSupport',struct('DataFileSelectedMaster',0,'DataFileSelectedLocal',0,'DataFileName','','DataFileDate','','SelectedFile',['<no file selected>']),'Options',struct('StatusSelected',1,'TimeSelected',1,'DeltaTimeSelected',1,'BytePortSelected',0,'MessageLengthSelected',0,'TriggerPort',struct('Selected',0,'TriggerType','rising'),'UserCoding',struct('Selected',0,'InterfaceFile','UserDecodingFile','FcnName','UserDecodeFcn','InportSelected',0,'InportWidth',1,'OutportSelected',0,'OutportWidth',1),'EnablePortSelected',0,'SignalOnPortnameSelected',1,'UseRXService',0),'Message',struct('MsgOnBlocknameSelected',0,'MsgName',['RX Message'],'MsgIdFormat',0,'MsgId',100,'MsgLength',8,'NumSignals',1,'SampleTime',-1,'Signal',struct('SgnName',['RX signal'],'SgnStartBit',0,'SgnLength',8,'SgnType',0,'ModeValue',-1,'DataType',0,'SLDataType','SS_DOUBLE','ByteLayout',0,'Factor',1,'Offset',0,'Min',0,'Max',255,'SgnComment',{{}},'SgnUnit',''),'MsgIdNumFormat',0,'MsgComment',{{''}}),'Version',1.2,'general',struct('isFromLib',1)),'GroupId',struct('Group',{{'RTICAN'}},'No',1,'Behavior',{{'NAMECHANGE'}},'BlockType',{{'SINK'}},'NameChangeFlag',0),'SFcnRTICANMessage',struct('MsgType','RX','MsgName',['RX Message'],'MsgIdFormat','STD','MsgId',100,'MsgLength',8,'NumSignals',1,'SampleTime',-1,'Signal',struct('SgnName',['RX signal'],'SgnStartBit',0,'SgnLength',8,'SgnType','standard','ModeValue',-1,'DataType',['unsigned int'],'ByteLayout',['little endian'],'SLDataType','SS_DOUBLE','Factor',1,'Offset',0),'StatusSelected','yes','TimeSelected','yes','DeltaTimeSelected','yes','BytePortSelected','no','MessageLengthSelected','no','EnablePortSelected','no','UserCoding',struct('Selected','no','InterfaceFile','UserDecodingFile','FcnName','UserDecodeFcn','InportSelected','no','InportWidth',1,'OutportSelected','no','OutportWidth',1),'TriggerPort',struct('Selected','no','TriggerType','rising'),'UseRXService','no','BoardType','DS4302','BoardNo',1,'ControllerNo',1,'SFcnPortType','Scalar'),'TLCFileName','rtican_rx_message')
      settings: AttributesFormatString=Group Id: RTICAN1\n  SourceProductName=dSPACE RTI CAN Blockset
  clock_time : Clock
  sub_time : Sum  Inputs=+-
  ROLL_bus : Outport  PortName=signals  Element=ROLL
  PITCH_bus : Outport  PortName=signals  Element=PITCH
  YAW_bus : Outport  PortName=signals  Element=YAW
  status : Outport  Port=2
  time : Outport  Port=3
  delta : Outport  Port=4
  wires:
  clock_time/1 -> sub_time/1
  sub_time/1 -> time/1
  SBG_ECAN_MSG_EKF_EULER1/4 -> status/1
  SBG_ECAN_MSG_EKF_EULER1/5 -> sub_time/2
  SBG_ECAN_MSG_EKF_EULER1/6 -> delta/1
  SBG_ECAN_MSG_EKF_EULER1/1 -> ROLL_bus/1  "ROLL"
  SBG_ECAN_MSG_EKF_EULER1/2 -> PITCH_bus/1  "PITCH"
  SBG_ECAN_MSG_EKF_EULER1/3 -> YAW_bus/1  "YAW"

== system dspace_2019/CAN RX/SBG_ECAN_MSG_EKF_INFO ==
  SBG_ECAN_MSG_EKF_INFO1 : rtican/RTICAN Receive (RX)   Reserved1=[]  Reserved2=[]  Reserved3=[]  Reserved4=[]  SfcnMessage=[]  Msg_Struct=[]  BoardTypeNo=[]  BoardNo=[]  ChannelNo=[]  Parameters=[]  DialogFcn=[]  UnitName=[]  Revision=[]  UnitValues=[]  DSProperties=struct('RTI',struct('Version',uint32(5),'BlockType',struct('isSLSource',uint8(1),'isSLSink',uint8(1),'isHWSource',uint8(0),'isHWSink',uint8(0),'isSetup',uint8(0),'isInline',uint8(1),'isNonInline',uint8(0),'isInterrupt',uint8(0),'isChannelwise',uint8(0)),'IOBoardType','RTICAN','UnitType','MESSAGE','Identifier','RX','DialogType','MSVC','BlockSet','RTICAN','SlaveProcessor','CAN'))  RTIBlockInterface=struct('OutputPortsWidth',int32([1 1 1 1]),'OutputPortsActive',[1 1 1 1],'OutputPortsName',{{'TIME_STAMP',['RX status'],['RX time'],['RX delta time']}},'OutputPortsDataType',{{'SS_DOUBLE','SS_DOUBLE','SS_DOUBLE','SS_DOUBLE'}},'OutputPortsLabel',{{'TIME_STAMP','','',''}},'OutputPortsLabelMode','ON','InputPortsWidth',int32(0),'InputPortsActive',0,'DialogFcn','rtican_message_interface_gui','BlockDisplay',{{'','center'}},'IconTransparency','on','ParameterTunableNames',{{}},'InitLevel',3,'BlockName',struct('Token',{{'SBG_ECAN_MSG_EKF_INFO'}}),'SampleTime',{{-1}},'TriggerPort',{{'none'}},'EnablePort',{{'none'}})  RTIBlockParameters=struct('BoardTypeNo',{{1,'OFF',[]}},'BoardNo',{{1,'ON',[1 16]}},'ChannelNo',{{2,'ON',[1 2]}},'Parameters',{{struct('DataFileSupport',struct('DataFileSelectedMaster',1,'DataFileSelectedLocal',1,'DataFileName','c:\users\oscar\documents\github\sw_infrastructure\kthfspe_python\databases\can1.dbc|','DataFileDate',{{{['10-Jul-2022 16:14:04']}}},'SelectedFile','c:\users\oscar\documents\github\sw_infrastructure\kthfspe_python\databases\can1.dbc'),'Options',struct('StatusSelected',1,'TimeSelected',1,'DeltaTimeSelected',1,'BytePortSelected',0,'MessageLengthSelected',0,'TriggerPort',struct('Selected',0,'TriggerType',0),'UserCoding',struct('Selected',0,'InterfaceFile','UserDecodingFile','FcnName','UserDecodeFcn','InportSelected',0,'InportWidth',1,'OutportSelected',0,'OutportWidth',1),'EnablePortSelected',0,'SignalOnPortnameSelected',1,'UseRXService',0),'Message',struct('MsgOnBlocknameSelected',1,'MsgName','SBG_ECAN_MSG_EKF_INFO','MsgIdFormat',0,'MsgId',304,'MsgLength',4,'NumSignals',1,'SampleTime',-1,'Signal',struct('SgnName','TIME_STAMP','SgnStartBit',0,'SgnLength',32,'SgnType',0,'ModeValue',-1,'DataType',0,'ByteLayout',0,'Factor',1,'Offset',0,'SgnComment',{{''}},'SgnUnit','ï¿½s','Min',0,'Max',2704,'SLDataType','SS_DOUBLE'),'MsgIdNumFormat',0,'MsgComment',{{''}}),'Version',1.2,'general',struct('isFromLib',0)),'OFF',[]}},'GroupId',{{struct('Group',{{'RTICAN'}},'No',1,'Behavior',{{'NAMECHANGE'}},'BlockType',{{'SINK'}},'NameChangeFlag',0),'OFF',[]}},'SFcnRTICANMessage',{{struct('MsgType','RX','SFcnPortType','Scalar','MsgName','SBG_ECAN_MSG_EKF_INFO','MsgIdFormat','STD','MsgId',304,'MsgLength',4,'NumSignals',1,'SampleTime',-1,'Signal',struct('SgnName','TIME_STAMP','SgnStartBit',0,'SgnLength',32,'SgnType','standard','ModeValue',-1,'DataType',['unsigned int'],'ByteLayout',['little endian'],'Factor',1,'Offset',0,'SLDataType','SS_DOUBLE'),'StatusSelected','yes','TimeSelected','yes','DeltaTimeSelected','yes','BytePortSelected','no','MessageLengthSelected','no','TriggerPort',struct('Selected','no','TriggerType',0),'UserCoding',struct('Selected','no','InterfaceFile','UserDecodingFile','FcnName','UserDecodeFcn','InportSelected','no','InportWidth',1,'OutportSelected','no','OutportWidth',1),'EnablePortSelected','no','UseRXService','no','BoardType','DS1','BoardNo',1,'ControllerNo',1),'OFF',[]}},'TLCFileName',{{'rtican_rx_message','OFF',[]}})  RTISFcnParameters=struct('SFcnRTICANMessage','struct','TLCFileName','char')  RTIBlockParaDefault=struct('BoardTypeNo',4302,'BoardNo',1,'ChannelNo',1,'Parameters',struct('DataFileSupport',struct('DataFileSelectedMaster',0,'DataFileSelectedLocal',0,'DataFileName','','DataFileDate','','SelectedFile',['<no file selected>']),'Options',struct('StatusSelected',1,'TimeSelected',1,'DeltaTimeSelected',1,'BytePortSelected',0,'MessageLengthSelected',0,'TriggerPort',struct('Selected',0,'TriggerType','rising'),'UserCoding',struct('Selected',0,'InterfaceFile','UserDecodingFile','FcnName','UserDecodeFcn','InportSelected',0,'InportWidth',1,'OutportSelected',0,'OutportWidth',1),'EnablePortSelected',0,'SignalOnPortnameSelected',1,'UseRXService',0),'Message',struct('MsgOnBlocknameSelected',0,'MsgName',['RX Message'],'MsgIdFormat',0,'MsgId',100,'MsgLength',8,'NumSignals',1,'SampleTime',-1,'Signal',struct('SgnName',['RX signal'],'SgnStartBit',0,'SgnLength',8,'SgnType',0,'ModeValue',-1,'DataType',0,'SLDataType','SS_DOUBLE','ByteLayout',0,'Factor',1,'Offset',0,'Min',0,'Max',255,'SgnComment',{{}},'SgnUnit',''),'MsgIdNumFormat',0,'MsgComment',{{''}}),'Version',1.2,'general',struct('isFromLib',1)),'GroupId',struct('Group',{{'RTICAN'}},'No',1,'Behavior',{{'NAMECHANGE'}},'BlockType',{{'SINK'}},'NameChangeFlag',0),'SFcnRTICANMessage',struct('MsgType','RX','MsgName',['RX Message'],'MsgIdFormat','STD','MsgId',100,'MsgLength',8,'NumSignals',1,'SampleTime',-1,'Signal',struct('SgnName',['RX signal'],'SgnStartBit',0,'SgnLength',8,'SgnType','standard','ModeValue',-1,'DataType',['unsigned int'],'ByteLayout',['little endian'],'SLDataType','SS_DOUBLE','Factor',1,'Offset',0),'StatusSelected','yes','TimeSelected','yes','DeltaTimeSelected','yes','BytePortSelected','no','MessageLengthSelected','no','EnablePortSelected','no','UserCoding',struct('Selected','no','InterfaceFile','UserDecodingFile','FcnName','UserDecodeFcn','InportSelected','no','InportWidth',1,'OutportSelected','no','OutportWidth',1),'TriggerPort',struct('Selected','no','TriggerType','rising'),'UseRXService','no','BoardType','DS4302','BoardNo',1,'ControllerNo',1,'SFcnPortType','Scalar'),'TLCFileName','rtican_rx_message')
      settings: AttributesFormatString=Group Id: RTICAN1\n  SourceProductName=dSPACE RTI CAN Blockset
  clock_time : Clock
  sub_time : Sum  Inputs=+-
  TIME_STAMP_bus : Outport  PortName=signals  Element=TIME_STAMP
  status : Outport  Port=2
  time : Outport  Port=3
  delta : Outport  Port=4
  wires:
  clock_time/1 -> sub_time/1
  sub_time/1 -> time/1
  SBG_ECAN_MSG_EKF_INFO1/2 -> status/1
  SBG_ECAN_MSG_EKF_INFO1/3 -> sub_time/2
  SBG_ECAN_MSG_EKF_INFO1/4 -> delta/1
  SBG_ECAN_MSG_EKF_INFO1/1 -> TIME_STAMP_bus/1  "TIME_STAMP"
